simulink model "garmi_whole_body_control"  (R2022a)
settings: Solver=ode1  StartTime=0.0  StopTime=5  FixedStep=.001  RelTol=1e-3  AbsTol=1e-3
libraries: simulink x1
settings Model: Creator=ge85xev  LastModifiedBy=ge85xev
settings SolverCC: AutoScaleAbsTol=off

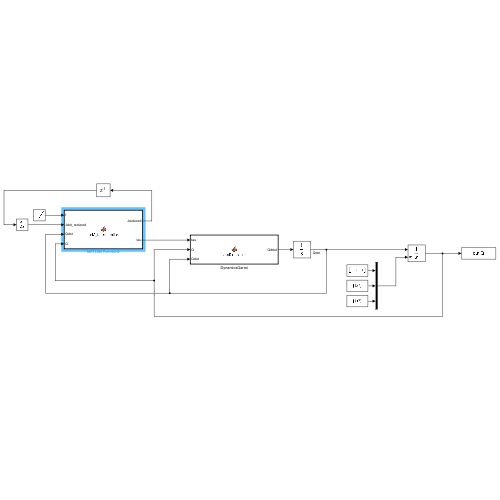
[thumbnail: Simulink's stored preview of the top-level diagram]
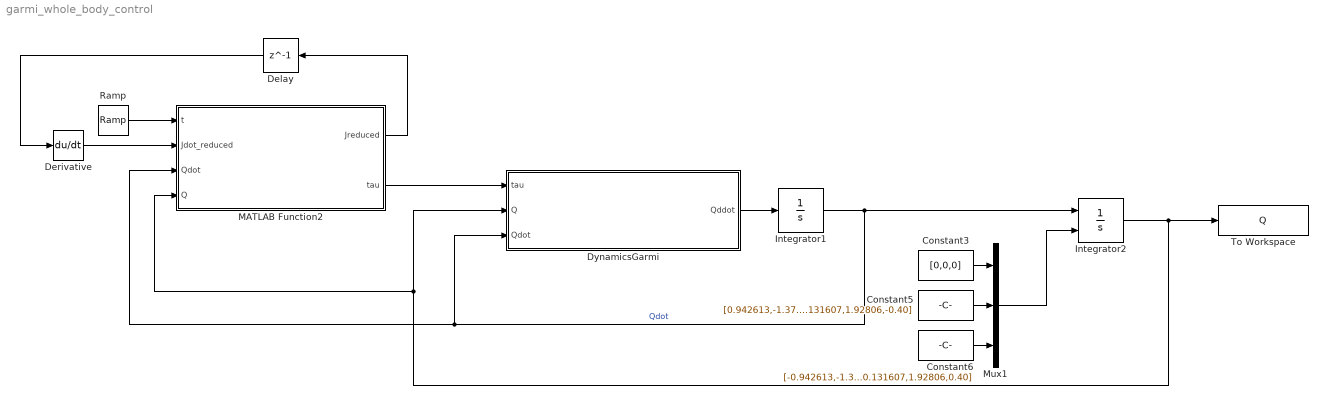
== system garmi_whole_body_control ==
  Constant3 : Constant  Value=[0,0,0]
  Constant5 : Constant  Value=[0.942613,-1.37299,-0.0288793,-1.84589,0.131607,1.92806,-0.40]
  Constant6 : Constant  Value=[-0.942613,-1.37299,-0.0288793,-1.84589,-0.131607,1.92806,0.40]
  Delay : Delay  DelayLength=1  InitialCondition=zeros(12,16)
  Derivative : Derivative
  DynamicsGarmi : MATLAB Function  TreatAsAtomicUnit=on  SystemSampleTime=0.001
  Integrator1 : Integrator  InitialCondition=[0,0,0,0,0,0,0,0,0,0,0,0,0,0,0,0,0]
  Integrator2 : Integrator  InitialConditionSource=external  InitialCondition=[0.942613,-1.37299,-0.0288793,-1.84589,0.131607,1.92806,-0.40]
  MATLAB Function2 : MATLAB Function  TreatAsAtomicUnit=on
  Mux1 : Mux  Inputs=3
  Ramp : simulink/Sources/Ramp  slope=1  start=0  InitialOutput=0
  To Workspace : ToWorkspace  VariableName=Q  SaveFormat=Timeseries  SampleTime=-1
  wires:
  Integrator1/1 -> DynamicsGarmi/3(Qdot), MATLAB Function2/3(Qdot), Integrator2/1  "Qdot"
  Integrator2/1 -> To Workspace/1, DynamicsGarmi/2(Q), MATLAB Function2/4(Q)
  Mux1/1 -> Integrator2/2
  Constant3/1 -> Mux1/1
  Constant5/1 -> Mux1/2
  Constant6/1 -> Mux1/3
  Derivative/1 -> MATLAB Function2/2(Jdot_reduced)
  MATLAB Function2/1(Jreduced) -> Delay/1
  Delay/1 -> Derivative/1
  Ramp/1 -> MATLAB Function2/1(t)
  DynamicsGarmi/1(Qddot) -> Integrator1/1
  MATLAB Function2/2(tau) -> DynamicsGarmi/1(tau)

== matlab function garmi_whole_body_control/MATLAB Function2 ==
  data: t input; Jdot_reduced input; Jreduced output; Qdot input; Q input; tau output
function  [Jreduced, tau] = arM_taskontroller(t,Jdot_reduced, Qdot, Q)
% Define control parameters for task space
% Define gains for translation and orientation components

K_task_translation = 30; % Stiffness for translation components
K_task_orientation = 10; % Stiffness for orientation components

D_task_translation = 10; % Damping for translation components
D_task_orientation = 4; % Damping for orientation components

% Create diagonal matrices for K_task, and D_task
% Including both translation and orientation components
K_task = diag([repmat(K_task_translation, 1, 3), repmat(K_task_orientation, 1, 3)]);
D_task = diag([repmat(D_task_translation, 1, 3), repmat(D_task_orientation, 1, 3)]);

% Define base, right arm, and left arm gains
K_null_base = 10; % Gain for the base
D_null_base = 45; % Damping for the base

% Gains for the right arm
K_null_right_arm = 1; % Example value, adjust as needed
D_null_right_arm = 1; % Example value, adjust as needed

% Gains for the left arm
K_null_left_arm = 1; % Example value, adjust as needed (can be different from right arm if desired)
D_null_left_arm = 1; % Example value, adjust as needed (can be different from right arm if desired)

% Create diagonal matrices for K_null and D_null
K_null = diag([repmat(K_null_base, 1, 3), ...
    repmat(K_null_right_arm, 1, 7), ...
    repmat(K_null_left_arm, 1, 7)]);

D_null = diag([repmat(D_null_base, 1, 3), ...
    repmat(D_null_right_arm, 1, 7), ...
    repmat(D_null_left_arm, 1, 7)]);

% Home positions for base and both arms
pose_base_home = [0.0,0,0]';
qhome_right = [0.942613,-1.37299,-0.0288793,-1.84589,0.131607,1.92806,-0.40]';
qhome_left = [-0.942613,-1.37299,-0.0288793,-1.84589,-0.131607,1.92806,0.40]'; % Example values, adjust as needed
Q_home = [pose_base_home;qhome_right;qhome_left];
Qdot_home = zeros(17,1);

% Compute whole body dynamics  model for the model based control.
[M, C, G] = computeDynamics(Q, Qdot);

% watch this video to learn how to drive these equations:
%  https://www.youtube.com/watch?v=C1cb03fYkxk

% Nonholomonic contriant matrix:
A = [-sin(Q(3)), cos(Q(3)), 0, zeros(1,14)];
Adot = [-Qdot(3)*cos(Q(3)), -Qdot(3)*sin(Q(3)), 0, zeros(1,14)];

% Computations for reduced order dynamics considering 1DOF nonholonomic
% dynamics
D = [cos(Q(3)), sin(Q(3)), zeros(1,15);zeros(15,2),eye(15,15)]; % D is auxilary and arbitrary matrix to make a non-singular square constriant matrix
Ddot = [-Qdot(3)*sin(Q(3)), Qdot(3)*cos(Q(3)), zeros(1,15);zeros(15,2),zeros(15,15)];
A_D = [A;D]; % This square matrix will be used to reduce the dynamics due to its constriant.
inverse_A_D = [-sin(Q(3)), cos(Q(3)), zeros(1,15);cos(Q(3)), sin(Q(3)), zeros(1,15);zeros(15,2),eye(15,15)]; % since the D matrix is easy, we analatically inverse it
E = inverse_A_D(:,1); % if the number of the constraints are M, then the first M columns are E
F = inverse_A_D(:,2:end); % if the number of the constraints are M, then the rest of columns (N-M) are F
v = D * Qdot;  % pseudo velocities that are used as the reduced generalized coordinates of the system.

% Compute Whole Body Jacobian for right and left arm
Jwb_right = JacobianWholeBody(Q,8,true);
Jwb_left = JacobianWholeBody(Q,8,false);

% Compute for pose of end effector for both right and left arms
pose_base_ref = [0;0;0];
Q_ref = [pose_base_ref;Q_home(4:17)]; % build Q_ref based on initial position of the base and q_home right and left arms
X_ref = [pose_arm(Q_ref, 8, true), pose_arm(Q_ref, 8, false)];
X = [pose_arm(Q, 8, true), pose_arm(Q, 8, false)];

Xdot_ref = [Jwb_right*zeros(17,1), Jwb_left*zeros(17,1)];
Xdot = [Jwb_right*Qdot, Jwb_left*Qdot];

% Compute for both right and left arms in one command.
u_task = zeros(16,2);
u_null = zeros(16,2);
Jreduced = [Jwb_right*F; Jwb_left*F];
M_reduced = F'*M*F; % Reduced mass matrix of the system.
M_reduced_inv = inv(M_reduced);

for arm_id = 1:2
    % task space
    Jr = Jreduced(6*arm_id-5:6*arm_id,:);
    Jd_r = Jdot_reduced(6*arm_id-5:6*arm_id,:);
    lambda = Jr * M_reduced_inv * Jr'; % auxilary variable that stores inverse of M_task. 
    M_task = inv(lambda);
    Jr_plus = Jr' / (Jr * Jr'); % compute pseudo inverse of Jr
    Jr_plus_M = M_reduced_inv * Jr' * M_task; % compute weighted pseudo inverse
    F_task = lambda * (K_task*(X_ref(:,arm_id) - X(:,arm_id)) + D_task*(Xdot_ref(:,arm_id) - Xdot(:,arm_id)));
    u_task(:,arm_id) = M_reduced*Jr_plus_M*(F_task - Jd_r*v);

    % null space
    Nr = eye(16) - Jr_plus_M*Jr; % compute null space.
    u_null(:,arm_id) = Nr'*F'*(K_null*(Q_home - Q) + D_null*(Qdot_home - Qdot));
end

F_p_pseudo = F / (F' * F);  % pseudo inverse of F';
u = u_task(:,1) + u_task(:,2) + u_null(:,1) + u_null(:,2);
%tau = (C*Qdot + G - M*(E*Adot + F*Ddot)*F*v) + F_p_pseudo*u + [20*(t<2.5);0;0;zeros(14,1)];
tau = (C*Qdot + G - M*(E*Adot + F*Ddot)*F*v) + F_p_pseudo*u + [40*(t<1);0;30*(t>2.0 && t<3);zeros(14,1)];
%tau = (C*Qdot + G - M*(E*Adot + F*Ddot)*F*v) + F_p_pseudo*u + Jwb_right'*[-15*(t<2);0;0;zeros(3,1)] + Jwb_left'*[-15*(t>2.5);0;0;zeros(3,1)];

% Compute reduced dynamics
%vdot = M_reduced_inv * F'*(tau - C*F*v - G + M*(E*Adot + F*Ddot)*F*v);  % reduced dynamics of the system.
%lambda_reduced = E'*(M*F*vdot - M*(E*Adot + F*Ddot)*F*v + C*Qdot + G - tau);  % reduced constraint forces.
%Qddot = F*vdot - (E*Adot + F*Ddot)*F*v;  % convert the reduced coordinates to the origin generalized coordinate.


    function crossMatrix = crossOperator(vec)
        crossMatrix = [0, -vec(3), vec(2); vec(3), 0, -vec(1); -vec(2), vec(1), 0];
    end

    function T = DHmatrix(q, i)
        % Define DH parameters for each link
        l = 0.1; % Tool length
        d = [0.333, 0, 0.316, 0, 0.384, 0, 0, 0.107+l];
        a = [0, 0, 0, 0.0825, -0.0825, 0, 0.088, 0];
        alpha = [0, -pi/2, pi/2, pi/2, -pi/2, pi/2, pi/2, 0];
        q_ext = [q; 0];

        % DH Transformation matrix for the current joint
        ct = cos(q_ext(i));
        st = sin(q_ext(i));
        ca = cos(alpha(i));
        sa = sin(alpha(i));

        T = [ ct, -st, 0, a(i);
            st * ca, ct * ca, -sa, -sa * d(i);
            st * sa, ct * sa, ca, ca * d(i);
            0, 0, 0, 1];  % calculate denavit hartenberg matrix
    end

    function T_total = FK(Q, index, isRightArm)
        % Extract pose components
        x = Q(1);
        y = Q(2);
        theta = Q(3);

        % Select the correct segment of Q based on isRightArm
        if isRightArm
            q_arm = Q(4:10); % Right arm joint angles
        else
            q_arm = Q(11:17); % Left arm joint angles
        end

        % --- Parameters Definition ---
        % Base dimensions
        width = 0.75; % X-direction (width)
        height = 0.2; % Y-direction (height)
        depth = 0.75; % Z-direction (depth)

        % Wheel parameters
        wheelRadius = height / 2; % Radius of the wheels

        % Spine length along the Z-axis and offset along the Y-axis
        spineHeight = 1.05;
        spineOffset = 0.1;

        % Shoulder width along the X-axis
        shoulderWidth = 0.4;

        % Rotation matrix to compensate the installation of Franka Arms on Garmi
        % torso
        if isRightArm
            beta = pi/2.0; % Rotation about Y axis
            gamma = pi/2.0; % Rotation about Z axis
            shoulderPose = [spineOffset , -shoulderWidth/2, height+ spineHeight]; % shoulderWidth/2 m to the right
        else
            beta = pi/2.0; % Rotation about Y axis
            gamma = -pi/2.0; % Rotation about Z axis
            shoulderPose = [spineOffset  , shoulderWidth/2, height+ spineHeight]; % shoulderWidth/2 m to the left
        end

        % Transformation matrix for the base of garmi
        T_mobile_base = [cos(theta), -sin(theta), 0 , x;
            sin(theta), cos(theta) , 0 , y;
            0,          0,           1 , 0;
            0,          0,           0 ,1];
        % Transformation matrix for the shoulder pose
        Tshoulder = [1, 0, 0, shoulderPose(1);
            0, 1, 0, shoulderPose(2);
            0, 0, 1, shoulderPose(3);
            0, 0, 0, 1];

        % Transformation matrix for the Garmi wall-mount arm installation
        Ty = [cos(beta), 0, sin(beta), 0;
            0, 1, 0, 0;
            -sin(beta), 0, cos(beta), 0;
            0, 0, 0, 1];
        Tz = [cos(gamma), -sin(gamma), 0, 0;
            sin(gamma), cos(gamma), 0, 0;
            0, 0, 1, 0;
            0, 0, 0, 1];

        % Transformation of the arm_base to the universal frame
        Ti = T_mobile_base* Tshoulder * Ty * Tz;

        for arm_id = 1:index
            Ti = Ti * DHmatrix(q_arm, arm_id); % apply rotation matrix to compensate for arm configuration
        end

        T_total = Ti;
    end

    function X = pose_arm(Q, index, isRightArm)
        % init pose vector:
        X = zeros(6,1);

        % Compute the transformation matrix for the specified configuration
        T_idx = FK(Q, index, isRightArm);

        % Extract the rotation matrix from the transformation matrix
        R = T_idx(1:3, 1:3);

        % Convert the rotation matrix to an axis-angle representation
        angle = acos((trace(R) - 1) / 2);
        if angle ~= 0
            % Ensure the angle is non-zero to avoid division by zero
            axis = [R(3,2) - R(2,3); R(1,3) - R(3,1); R(2,1) - R(1,2)] / (2*sin(angle));
            % Normalize the axis to ensure it's a unit vector
            axis = axis / norm(axis);
        else
            % Handle the case of a zero angle, implying no rotation or a full rotation
            axis = [0; 0; 1]; % Default axis if no rotation is present
        end

        % return pose vector
        X(1:3)= T_idx(1:3,4);
        X(4:6) = angle * axis;
    end

    function positions = getJointsPositions(Q, isRightArm)
        positions = zeros(3, 8); % Initialize positions matrix

        for arm_id = 1:8
            T = FK(Q, arm_id, isRightArm);
            positions(:, arm_id) = T(1:3, 4); % Extract and store the position
        end
    end

    function Jacobian = JacobArm(Q, index, isRightArm)

        % Initialize the Jacobian matrix with zeros
        Jacobian = zeros(6, 7);

        % Compute FK up to the specified joint index
        T_joint_index = FK(Q, index, isRightArm);
        P_joint_index = T_joint_index(1:3, 4); % Extract the position vector of the joint at the specified index

        for arm_id = 1:index-1  % count joint positions up to one before the target joint.
            % Compute the transformation matrix up to the current joint
            Ti = FK(Q, arm_id, isRightArm);

            % Extract the joint axis of the current joint
            P_i = Ti(1:3, 4);

            % Calculate the columns of the Jacobian matrix
            z_current = Ti(1:3, 3);
            p_diff = P_joint_index - P_i;

            % Update the Jacobian matrix
            % Linear velocity part
            Jacobian(1:3, arm_id) = cross(z_current, p_diff);
            % Angular velocity part
            Jacobian(4:6, arm_id) = z_current;
        end
    end

    function Jacobian = JacobBody(Q, index, isRightArm)

        % Compute FK up to the specified joint index
        T_joint_index = FK(Q, index, isRightArm);

        % Extract the position of the joint at the specified index
        % in absolute frame relative to robot base center.
        P_joint_index = T_joint_index(1:3, 4) - [Q(1),Q(2),0]';

        % Nonholonomic matrix setup (assuming linear and angular velocity command scenario)
        nonholonomicMatrix = [1, 0, 0 ; 0, 1, 0 ; 0, 0, 0 ; 0, 0, 0 ; 0, 0, 0 ; 0, 0, 1];
        %nonholonomicMatrix = [cos(pose(3)), 0; sin(pose(3)), 0; 0, 0; 0, 0; 0, 0; 0, 1];

        % Calculate the Jacobian for the platform
        crossProdMatrix = crossOperator(P_joint_index);
        JacobianPlatform = [eye(3), -crossProdMatrix; zeros(3, 3), eye(3)];

        % Apply the nonholonomic constraints to the platform Jacobian
        Jacobian = JacobianPlatform * nonholonomicMatrix;
    end

    function J_wb = JacobianWholeBody(Q, index, isRightArm)
        J_arm = JacobArm(Q, index, isRightArm);
        J_body = JacobBody(Q, index, isRightArm);
        if isRightArm
            % Assemble the whole-body Jacobian for the right side
            J_wb = [J_body, J_arm, zeros(6, 7)];
        else
            % Assemble the whole-body Jacobian for the left side
            J_wb = [J_body, zeros(6, 7), J_arm];
        end
    end

    function jacobian = JacobArm_cg(Q, index, isRightArm)
        jacobian = zeros(6, 7); % Pre-allocate for speed
        linkCoMs = zeros(3, 7);

        % Updated CoM for each link (expressed as offsets from the link frame)
        linkCoMs = [0, -0.0256, 0.00652, -0.0472, -0.00402, 0.1263, 0.1;
            -5.844e-9, -0.323, 0.0228, 0.000919, 0.0770, -0.0410, 0.00290;
            -0.391, 0.0706, -0.0701, 0.0287, -0.376, -0.0109, 0.0272];

        T_mi = FK(Q, index, isRightArm);
        R_mi = T_mi(1:3,1:3);
        joint_position_before_mi = T_mi(1:3,4);
        r_mi_abs = joint_position_before_mi + R_mi * linkCoMs(:, index); % center of mass position of link i in global frame relative to global frame

        for joint_number = 1:index
            Ti = FK(Q,joint_number,isRightArm);
            joint_position = Ti(1:3,4);
            joint_axis = Ti(1:3,3);  % frame z axis is equivalent to the joint axis vector.

            jacobian(1:3, joint_number) = cross(joint_axis, (r_mi_abs - joint_position));
            jacobian(4:6, joint_number) = joint_axis;
        end
    end

    function Jacobian = JacobBody_cg(Q, index, isRightArm)

        % Updated CoM for each link (expressed as offsets from the link frame)
        linkCoMs = [0, -0.0256, 0.00652, -0.0472, -0.00402, 0.1263, 0.1;
            -5.844e-9, -0.323, 0.0228, 0.000919, 0.0770, -0.0410, 0.00290;
            -0.391, 0.0706, -0.0701, 0.0287, -0.376, -0.0109, 0.0272];

        % Compute FK up to the specified joint index
        T_mi = FK(Q, index, isRightArm);
        R_mi = T_mi(1:3,1:3);
        joint_position_before_cg = T_mi(1:3,4);
        r_mi_abs = joint_position_before_cg + R_mi * linkCoMs(:, index); % center of mass position of link i in global frame


        r_mi_abs_rel = r_mi_abs - [Q(1),Q(2),0]'; % center of mass position of link i relative to mobile base frame

        % Nonholonomic matrix setup (assuming linear and angular velocity command scenario)
        nonholonomicMatrix = [1, 0, 0 ; 0, 1, 0 ; 0, 0, 0 ; 0, 0, 0 ; 0, 0, 0 ; 0, 0, 1];

        % Calculate the Jacobian for the platform
        crossProdMatrix = crossOperator(r_mi_abs_rel);
        JacobianPlatform = [eye(3), -crossProdMatrix; zeros(3, 3), eye(3)];

        % Apply the nonholonomic constraints to the platform Jacobian
        Jacobian = JacobianPlatform * nonholonomicMatrix;
    end

    function J_wb = JacobianWholeBody_cg(Q, index, isRightArm)
        J_arm = JacobArm_cg(Q, index, isRightArm);
        J_body = JacobBody_cg(Q, index, isRightArm);
        if isRightArm
            % Assemble the whole-body Jacobian for the right side
            J_wb = [J_body, J_arm, zeros(6, 7)];
        else
            % Assemble the whole-body Jacobian for the left side
            J_wb = [J_body, zeros(6, 7), J_arm];
        end
    end

% Dynamics
    function [M, C, G] = computeDynamics(Q, Qdot)
        % Dynamic parameters
        g = [0; 0; -9.81];

        % Updated mass for each link
        linkMasses = [4.07, 5.996, 0.570, 3.083, 3.616, 1.435, 0.453];

        % Updated inertia matrices for each link, approximated and written inline
        linkInertia = zeros(3, 21);
        linkInertia(:, 1:3) = [4.47e-6, 0, 0; 0, 4.47e-6, -5.61e-10; 0, -5.61e-10, 2.00e-6]; % Link 1
        linkInertia(:, 4:6) = [0.0465, -0.00338, 0.000748; -0.00338, 0.00243, 0.00980; 0.000748, 0.00980, 0.0445]; % Link 2
        linkInertia(:, 7:9) = [0.0504, 0.00248, -0.0118; 0.00248, 0.0525, 0.00747; -0.0118, 0.00747, 0.00817]; % Link 3
        linkInertia(:, 10:12) = [0.0308, 0.00732, 0.000194; 0.00732, 0.00278, 0.00101; 0.000194, 0.00101, 0.0329]; % Link 4
        linkInertia(:, 13:15) = [0.0511, -0.000984, -0.00223; -0.000984, 0.0472, 0.00346; -0.00223, 0.00346, 0.00475]; % Link 5
        linkInertia(:, 16:18) = [0.00823, 0.00463, -0.00127; 0.00463, 0.0187, 0.00110; -0.00127, 0.00110, 0.0144]; % Link 6
        linkInertia(:, 19:21) = [0.00378, -3.27e-5, -0.000200; -3.27e-5, 0.00368, -0.000602; -0.000200, -0.000602, 0.000122]; % Link 7


        % Mass and Inertia parameters for mobile base
        baseMass = 10;
        baseInertia = 3;

        M = zeros(17, 17);
        C = zeros(17, 17);
        G = zeros(17, 1);

        % Arm dynamics computation for both arms
        for arm = 1:2 % 1 for right arm, 2 for left arm
            for arm_id = 1:7
                Tcg = FK(Q, arm_id, arm == 1);
                Rcg = Tcg(1:3, 1:3);
                Jwb_cg = JacobianWholeBody_cg(Q, arm_id, arm == 1);
                linkmass = linkMasses(arm_id);
                InertiaMatrix = reshape(linkInertia(:, 3*arm_id-2:3*arm_id), 3, 3);

                mass_link = zeros(6, 6);
                mass_link(1:3, 1:3) = linkmass * eye(3);
                mass_link(4:6, 4:6) = Rcg * InertiaMatrix * Rcg';

                Jwb_cg_v = Jwb_cg(1:3, :);

                M = M + Jwb_cg' * mass_link * Jwb_cg;
                G = G - linkmass * Jwb_cg_v' * g;
            end
            C = zeros(17, 1);
        end

        JacobBase = [eye(3),zeros(3,7),zeros(3,7)];  % jacobian of mobile base vb = JacobBase*Qdot
        % Base dynamics
        M = M + JacobBase'*diag([baseMass, baseMass, baseInertia])*JacobBase;
        G = G + zeros(17,1);
        C = C + zeros(17, 17);
    end
end

== matlab function garmi_whole_body_control/DynamicsGarmi ==
  data: tau input; Q input; Qdot input; Qddot output
function Qddot  = stepSimulation(tau, Q, Qdot)
% Check the norm of the joint angles for both arms
if norm(Q(1:7)) > 10 || norm(Q(8:end)) > 10
    disp('The simulation has diverged.');
end

% Compute the dynamics of the robot. In real experiment scenarios, this
% step will be done by the physics
[M, C, G] = computeDynamics(Q, Qdot);

% Nonholomonic contriant matrix:
A = [-sin(Q(3)), cos(Q(3)), 0, zeros(1,14)];
Adot = [-Qdot(3)*cos(Q(3)), -Qdot(3)*sin(Q(3)), 0, zeros(1,14)];
A_M_pseudo = (M \ A') / (A * (M \ A'));  % Weighted (M) pseudo inverse of A matrix

% calculate lambda multiplier for the nonholonomic constraint (basic method):
lambda = (A_M_pseudo)'*(C * Qdot + G - tau) - (A / M * A')\ Adot * Qdot;

% Solve for dynamics equation with the presence of nonholonomic constriant.
Qddot = M \ (-C * Qdot - G + tau + A'*lambda);

% I embeded the lambda in the dynamics equation as discussed in the video.
% The results would be the following equation:
% Qddot = M \ ((eye(17,17) - Aq'*A_M_pseudo')*(tau - C*Qdot - G) - M * A_M_pseudo*Aqdot*Qdot);

    function crossMatrix = crossOperator(vec)
        crossMatrix = [0, -vec(3), vec(2); vec(3), 0, -vec(1); -vec(2), vec(1), 0];
    end

    function T = DHmatrix(q, i)
        % Define DH parameters for each link
        l = 0.1; % Tool length
        d = [0.333, 0, 0.316, 0, 0.384, 0, 0, 0.107+l];
        a = [0, 0, 0, 0.0825, -0.0825, 0, 0.088, 0];
        alpha = [0, -pi/2, pi/2, pi/2, -pi/2, pi/2, pi/2, 0];
        q_ext = [q; 0];

        % DH Transformation matrix for the current joint
        ct = cos(q_ext(i));
        st = sin(q_ext(i));
        ca = cos(alpha(i));
        sa = sin(alpha(i));

        T = [ ct, -st, 0, a(i);
            st * ca, ct * ca, -sa, -sa * d(i);
            st * sa, ct * sa, ca, ca * d(i);
            0, 0, 0, 1];  % calculate denavit hartenberg matrix
    end

    function T_total = FK(Q, index, isRightArm)
        % Extract pose components
        x = Q(1);
        y = Q(2);
        theta = Q(3);

        % Select the correct segment of Q based on isRightArm
        if isRightArm
            q_arm = Q(4:10); % Right arm joint angles
        else
            q_arm = Q(11:17); % Left arm joint angles
        end

        % --- Parameters Definition ---
        % Base dimensions
        width = 0.75; % X-direction (width)
        height = 0.2; % Y-direction (height)
        depth = 0.75; % Z-direction (depth)

        % Wheel parameters
        wheelRadius = height / 2; % Radius of the wheels

        % Spine length along the Z-axis and offset along the Y-axis
        spineHeight = 1.05;
        spineOffset = 0.1;

        % Shoulder width along the X-axis
        shoulderWidth = 0.4;

        % Rotation matrix to compensate the installation of Franka Arms on Garmi
        % torso
        if isRightArm
            beta = pi/2.0; % Rotation about Y axis
            gamma = pi/2.0; % Rotation about Z axis
            shoulderPose = [spineOffset , -shoulderWidth/2, height+ spineHeight]; % shoulderWidth/2 m to the right
        else
            beta = pi/2.0; % Rotation about Y axis
            gamma = -pi/2.0; % Rotation about Z axis
            shoulderPose = [spineOffset  , shoulderWidth/2, height+ spineHeight]; % shoulderWidth/2 m to the left
        end

        % Transformation matrix for the base of garmi
        T_mobile_base = [cos(theta), -sin(theta), 0 , x;
            sin(theta), cos(theta) , 0 , y;
            0,          0,           1 , 0;
            0,          0,           0 ,1];
        % Transformation matrix for the shoulder pose
        Tshoulder = [1, 0, 0, shoulderPose(1);
            0, 1, 0, shoulderPose(2);
            0, 0, 1, shoulderPose(3);
            0, 0, 0, 1];

        % Transformation matrix for the Garmi wall-mount arm installation
        Ty = [cos(beta), 0, sin(beta), 0;
            0, 1, 0, 0;
            -sin(beta), 0, cos(beta), 0;
            0, 0, 0, 1];
        Tz = [cos(gamma), -sin(gamma), 0, 0;
            sin(gamma), cos(gamma), 0, 0;
            0, 0, 1, 0;
            0, 0, 0, 1];

        % Transformation of the arm_base to the universal frame
        Ti = T_mobile_base* Tshoulder * Ty * Tz;

        for arm_id = 1:index
            Ti = Ti * DHmatrix(q_arm, arm_id); % apply rotation matrix to compensate for arm configuration
        end

        T_total = Ti;
    end

    function X = pose_arm(Q, index, isRightArm)
        % init pose vector:
        X = zeros(6,1);

        % Compute the transformation matrix for the specified configuration
        T_idx = FK(Q, index, isRightArm);

        % Extract the rotation matrix from the transformation matrix
        R = T_idx(1:3, 1:3);

        % Convert the rotation matrix to an axis-angle representation
        angle = acos((trace(R) - 1) / 2);
        if angle ~= 0
            % Ensure the angle is non-zero to avoid division by zero
            axis = [R(3,2) - R(2,3); R(1,3) - R(3,1); R(2,1) - R(1,2)] / (2*sin(angle));
            % Normalize the axis to ensure it's a unit vector
            axis = axis / norm(axis);
        else
            % Handle the case of a zero angle, implying no rotation or a full rotation
            axis = [0; 0; 1]; % Default axis if no rotation is present
        end

        % return pose vector
        X(1:3)= T_idx(1:3,4);
        X(4:6) = angle * axis;
    end

    function positions = getJointsPositions(Q, isRightArm)
        positions = zeros(3, 8); % Initialize positions matrix

        for arm_id = 1:8
            T = FK(Q, arm_id, isRightArm);
            positions(:, arm_id) = T(1:3, 4); % Extract and store the position
        end
    end

    function Jacobian = JacobArm(Q, index, isRightArm)

        % Initialize the Jacobian matrix with zeros
        Jacobian = zeros(6, 7);

        % Compute FK up to the specified joint index
        T_joint_index = FK(Q, index, isRightArm);
        P_joint_index = T_joint_index(1:3, 4); % Extract the position vector of the joint at the specified index

        for arm_id = 1:index-1  % count joint positions up to one before the target joint.
            % Compute the transformation matrix up to the current joint
            Ti = FK(Q, arm_id, isRightArm);

            % Extract the joint axis of the current joint
            P_i = Ti(1:3, 4);

            % Calculate the columns of the Jacobian matrix
            z_current = Ti(1:3, 3);
            p_diff = P_joint_index - P_i;

            % Update the Jacobian matrix
            % Linear velocity part
            Jacobian(1:3, arm_id) = cross(z_current, p_diff);
            % Angular velocity part
            Jacobian(4:6, arm_id) = z_current;
        end
    end

    function Jacobian = JacobBody(Q, index, isRightArm)

        % Compute FK up to the specified joint index
        T_joint_index = FK(Q, index, isRightArm);

        % Extract the position of the joint at the specified index
        % in absolute frame relative to robot base center.
        P_joint_index = T_joint_index(1:3, 4) - [Q(1),Q(2),0]';

        % Nonholonomic matrix setup (assuming linear and angular velocity command scenario)
        nonholonomicMatrix = [1, 0, 0 ; 0, 1, 0 ; 0, 0, 0 ; 0, 0, 0 ; 0, 0, 0 ; 0, 0, 1];
        %nonholonomicMatrix = [cos(pose(3)), 0; sin(pose(3)), 0; 0, 0; 0, 0; 0, 0; 0, 1];

        % Calculate the Jacobian for the platform
        crossProdMatrix = crossOperator(P_joint_index);
        JacobianPlatform = [eye(3), -crossProdMatrix; zeros(3, 3), eye(3)];

        % Apply the nonholonomic constraints to the platform Jacobian
        Jacobian = JacobianPlatform * nonholonomicMatrix;
    end

    function J_wb = JacobianWholeBody(Q, index, isRightArm)
        J_arm = JacobArm(Q, index, isRightArm);
        J_body = JacobBody(Q, index, isRightArm);
        if isRightArm
            % Assemble the whole-body Jacobian for the right side
            J_wb = [J_body, J_arm, zeros(6, 7)];
        else
            % Assemble the whole-body Jacobian for the left side
            J_wb = [J_body, zeros(6, 7), J_arm];
        end
    end

    function jacobian = JacobArm_cg(Q, index, isRightArm)
        jacobian = zeros(6, 7); % Pre-allocate for speed
        linkCoMs = zeros(3, 7);

        % Updated CoM for each link (expressed as offsets from the link frame)
        linkCoMs = [0, -0.0256, 0.00652, -0.0472, -0.00402, 0.1263, 0.1;
            -5.844e-9, -0.323, 0.0228, 0.000919, 0.0770, -0.0410, 0.00290;
            -0.391, 0.0706, -0.0701, 0.0287, -0.376, -0.0109, 0.0272];

        T_mi = FK(Q, index, isRightArm);
        R_mi = T_mi(1:3,1:3);
        joint_position_before_mi = T_mi(1:3,4);
        r_mi_abs = joint_position_before_mi + R_mi * linkCoMs(:, index); % center of mass position of link i in global frame relative to global frame

        for joint_number = 1:index
            Ti = FK(Q,joint_number,isRightArm);
            joint_position = Ti(1:3,4);
            joint_axis = Ti(1:3,3);  % frame z axis is equivalent to the joint axis vector.

            jacobian(1:3, joint_number) = cross(joint_axis, (r_mi_abs - joint_position));
            jacobian(4:6, joint_number) = joint_axis;
        end
    end

    function Jacobian = JacobBody_cg(Q, index, isRightArm)

        % Updated CoM for each link (expressed as offsets from the link frame)
        linkCoMs = [0, -0.0256, 0.00652, -0.0472, -0.00402, 0.1263, 0.1;
            -5.844e-9, -0.323, 0.0228, 0.000919, 0.0770, -0.0410, 0.00290;
            -0.391, 0.0706, -0.0701, 0.0287, -0.376, -0.0109, 0.0272];

        % Compute FK up to the specified joint index
        T_mi = FK(Q, index, isRightArm);
        R_mi = T_mi(1:3,1:3);
        joint_position_before_cg = T_mi(1:3,4);
        r_mi_abs = joint_position_before_cg + R_mi * linkCoMs(:, index); % center of mass position of link i in global frame


        r_mi_abs_rel = r_mi_abs - [Q(1),Q(2),0]'; % center of mass position of link i relative to mobile base frame

        % Nonholonomic matrix setup (assuming linear and angular velocity command scenario)
        nonholonomicMatrix = [1, 0, 0 ; 0, 1, 0 ; 0, 0, 0 ; 0, 0, 0 ; 0, 0, 0 ; 0, 0, 1];

        % Calculate the Jacobian for the platform
        crossProdMatrix = crossOperator(r_mi_abs_rel);
        JacobianPlatform = [eye(3), -crossProdMatrix; zeros(3, 3), eye(3)];

        % Apply the nonholonomic constraints to the platform Jacobian
        Jacobian = JacobianPlatform * nonholonomicMatrix;
    end

    function J_wb = JacobianWholeBody_cg(Q, index, isRightArm)
        J_arm = JacobArm_cg(Q, index, isRightArm);
        J_body = JacobBody_cg(Q, index, isRightArm);
        if isRightArm
            % Assemble the whole-body Jacobian for the right side
            J_wb = [J_body, J_arm, zeros(6, 7)];
        else
            % Assemble the whole-body Jacobian for the left side
            J_wb = [J_body, zeros(6, 7), J_arm];
        end
    end

% Dynamics
    function [M, C, G] = computeDynamics(Q, Qdot)
        % Dynamic parameters
        g = [0; 0; -9.81];

        % Updated mass for each link
        linkMasses = [4.07, 5.996, 0.570, 3.083, 3.616, 1.435, 0.453];

        % Updated inertia matrices for each link, approximated and written inline
        linkInertia = zeros(3, 21);
        linkInertia(:, 1:3) = [4.47e-6, 0, 0; 0, 4.47e-6, -5.61e-10; 0, -5.61e-10, 2.00e-6]; % Link 1
        linkInertia(:, 4:6) = [0.0465, -0.00338, 0.000748; -0.00338, 0.00243, 0.00980; 0.000748, 0.00980, 0.0445]; % Link 2
        linkInertia(:, 7:9) = [0.0504, 0.00248, -0.0118; 0.00248, 0.0525, 0.00747; -0.0118, 0.00747, 0.00817]; % Link 3
        linkInertia(:, 10:12) = [0.0308, 0.00732, 0.000194; 0.00732, 0.00278, 0.00101; 0.000194, 0.00101, 0.0329]; % Link 4
        linkInertia(:, 13:15) = [0.0511, -0.000984, -0.00223; -0.000984, 0.0472, 0.00346; -0.00223, 0.00346, 0.00475]; % Link 5
        linkInertia(:, 16:18) = [0.00823, 0.00463, -0.00127; 0.00463, 0.0187, 0.00110; -0.00127, 0.00110, 0.0144]; % Link 6
        linkInertia(:, 19:21) = [0.00378, -3.27e-5, -0.000200; -3.27e-5, 0.00368, -0.000602; -0.000200, -0.000602, 0.000122]; % Link 7


        % Mass and Inertia parameters for mobile base
        baseMass = 10;
        baseInertia = 3;

        M = zeros(17, 17);
        C = zeros(17, 17);
        G = zeros(17, 1);

        % Arm dynamics computation for both arms
        for arm = 1:2 % 1 for right arm, 2 for left arm
            for arm_id = 1:7
                Tcg = FK(Q, arm_id, arm == 1);
                Rcg = Tcg(1:3, 1:3);
                Jwb_cg = JacobianWholeBody_cg(Q, arm_id, arm == 1);
                linkmass = linkMasses(arm_id);
                InertiaMatrix = reshape(linkInertia(:, 3*arm_id-2:3*arm_id), 3, 3);

                mass_link = zeros(6, 6);
                mass_link(1:3, 1:3) = linkmass * eye(3);
                mass_link(4:6, 4:6) = Rcg * InertiaMatrix * Rcg';

                Jwb_cg_v = Jwb_cg(1:3, :);

                M = M + Jwb_cg' * mass_link * Jwb_cg;
                G = G - linkmass * Jwb_cg_v' * g;
            end
            C = zeros(17, 1);
        end

        JacobBase = [eye(3),zeros(3,7),zeros(3,7)];  % jacobian of mobile base vb = JacobBase*Qdot
        % Base dynamics
        M = M + JacobBase'*diag([baseMass, baseMass, baseInertia])*JacobBase;
        G = G + zeros(17,1);
        C = C + zeros(17, 17);
    end

end
